simulink library "halout"  (R2021b)
settings: Solver=VariableStepAuto  StartTime=0.0  StopTime=10.0  RelTol=1e-3
undefined symbols (not defined in the file): C_TASK_5MS_S, KHAL_CAN1TxReq_flg, KHAL_CAN2TxReq_flg, KHAL_CAN3TxReq_flg, KHAL_CAN4TxReq_flg, KHAL_CAN5TxReq_flg, KHAL_CAN6TxReq_flg, KHAL_CAN7TxReq_flg, TRUE
libraries: FVT_lib x65, simulink x6
(part 3 of 6)

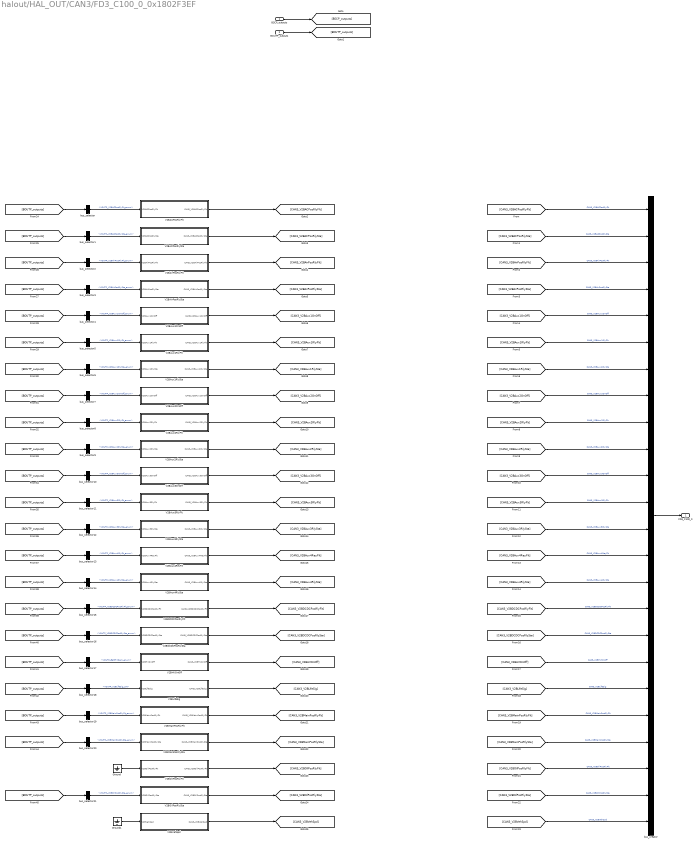
== system halout/HAL_OUT/CAN3/FD3_C100_0_0x1802F3EF ==
  BSCP_outputs : Inport  OutDataTypeStr=Bus: BSCP_outputs
  BOUTP_outputs : Inport  Port=2  OutDataTypeStr=Bus: BOUTP_outputs
  Ground : Ground
  Ground1 : Ground
  V2BACPosRlyFlt : Subsystem
  V2BACPosRlySta : Subsystem
  V2BAirPosRlyFlt : Subsystem
  V2BAirPosRlySta : Subsystem
  V2BAux1OnOff : Subsystem
  V2BAux1RlyFlt : Subsystem
  V2BAux1RlySta : Subsystem
  V2BAux2OnOff : Subsystem
  V2BAux2RlyFlt : Subsystem
  V2BAux2RlySta : Subsystem
  V2BAux3OnOff : Subsystem
  V2BAux3RlyFlt : Subsystem
  V2BAux3RlySta : Subsystem
  V2BAux4ReyFlt : Subsystem
  V2BAux4RlySta : Subsystem
  V2BDCDCPosRlyFlt : Subsystem
  V2BDCDCPosRlySta : Subsystem
  V2BHVOnOff : Subsystem
  V2BLifeSig : Subsystem
  V2BMainPosRlyFlt : Subsystem
  V2BMainPosRlySta : Subsystem
  V2BOilPosRlyFlt : Subsystem
  V2BOilPosRlySta : Subsystem
  V2BVehSpd : Subsystem
  bus_creator : BusCreator  Inputs=24  OutDataTypeStr=Bus: DT_CAN3_SG_FD3_C100_0  NonVirtualBus=on
  bus_selector : BusSelector  OutputSignals=VOUTP_V2BACPosRlyFit_enum
  bus_selector1 : BusSelector  OutputSignals=VOUTP_V2BACPosRlySta_enum
  bus_selector10 : BusSelector  OutputSignals=VOUTP_V2BAux3OnOff_enum
  bus_selector11 : BusSelector  OutputSignals=VOUTP_V2BAux3RlyFit_enum
  bus_selector12 : BusSelector  OutputSignals=VOUTP_V2BAux3RlySta_enum
  bus_selector13 : BusSelector  OutputSignals=VOUTP_V2BAux4RlyFit_enum
  bus_selector14 : BusSelector  OutputSignals=VOUTP_V2BAux4RlySta_enum
  bus_selector15 : BusSelector  OutputSignals=VOUTP_V2BDCDCPosRlyFit_enum
  bus_selector16 : BusSelector  OutputSignals=VOUTP_V2BDCDCPosRlySta_enum
  bus_selector17 : BusSelector  OutputSignals=VOUTP_BattHVDem_enum
  bus_selector18 : BusSelector  OutputSignals=VOUTP_V2BLifeSig_cnt
  bus_selector19 : BusSelector  OutputSignals=VOUTP_V2BMainPosRlyFit_enum
  bus_selector2 : BusSelector  OutputSignals=VOUTP_V2BAirPosRlyFit_enum
  bus_selector20 : BusSelector  OutputSignals=VOUTP_V2BMainPosRlySta_enum
  bus_selector21 : BusSelector  OutputSignals=VOUTP_V2BOilPosRlySta_enum
  bus_selector3 : BusSelector  OutputSignals=VOUTP_V2BAirPosRlySta_enum
  bus_selector4 : BusSelector  OutputSignals=VOUTP_V2BAux1OnOff_enum
  bus_selector5 : BusSelector  OutputSignals=VOUTP_V2BAux1RlyFit_enum
  bus_selector6 : BusSelector  OutputSignals=VOUTP_V2BAux1RlySta_enum
  bus_selector7 : BusSelector  OutputSignals=VOUTP_V2BAux2OnOff_enum
  bus_selector8 : BusSelector  OutputSignals=VOUTP_V2BAux2RlyFit_enum
  bus_selector9 : BusSelector  OutputSignals=VOUTP_V2BAux2RlySta_enum
  FD3_C100_0 : Outport
  wires:
  BSCP_outputs/1 -> [BSCP_outputs]
  BOUTP_outputs/1 -> [BOUTP_outputs]
  [CAN3_V2BACPosRlyFlt] -> bus_creator/1  "CAN3_V2BACPosRlyFlt"
  [CAN3_V2BACPosRlySta] -> bus_creator/2  "CAN3_V2BACPosRlySta"
  [CAN3_V2BAirPosRlyFlt] -> bus_creator/3  "CAN3_V2BAirPosRlyFlt"
  [CAN3_V2BAirPosRlySta] -> bus_creator/4  "CAN3_V2BAirPosRlySta"
  [CAN3_V2BAux1OnOff] -> bus_creator/5  "CAN3_V2BAux1OnOff"
  [CAN3_V2BAux1RlyFlt] -> bus_creator/6  "CAN3_V2BAux1RlyFlt"
  [CAN3_V2BAux1RlySta] -> bus_creator/7  "CAN3_V2BAux1RlySta"
  [CAN3_V2BAux2OnOff] -> bus_creator/8  "CAN3_V2BAux2OnOff"
  [CAN3_V2BAux2RlyFlt] -> bus_creator/9  "CAN3_V2BAux2RlyFlt"
  [CAN3_V2BAux2RlySta] -> bus_creator/10  "CAN3_V2BAux2RlySta"
  [CAN3_V2BAux3OnOff] -> bus_creator/11  "CAN3_V2BAux3OnOff"
  [CAN3_V2BAux3RlyFlt] -> bus_creator/12  "CAN3_V2BAux3RlyFlt"
  [CAN3_V2BAux3RlySta] -> bus_creator/13  "CAN3_V2BAux3RlySta"
  [CAN3_V2BAux4ReyFlt] -> bus_creator/14  "CAN3_V2BAux4ReyFlt"
  [CAN3_V2BAux4RlySta] -> bus_creator/15  "CAN3_V2BAux4RlySta"
  [CAN3_V2BDCDCPosRlyFlt] -> bus_creator/16  "CAN3_V2BDCDCPosRlyFlt"
  [CAN3_V2BDCDCPosRlySta] -> bus_creator/17  "CAN3_V2BDCDCPosRlySta"
  [CAN3_V2BHVOnOff] -> bus_creator/18  "CAN3_V2BHVOnOff"
  [CAN3_V2BLifeSig] -> bus_creator/19  "CAN3_V2BLifeSig"
  [CAN3_V2BMainPosRlyFlt] -> bus_creator/20  "CAN3_V2BMainPosRlyFlt"
  [CAN3_V2BMainPosRlySta] -> bus_creator/21  "CAN3_V2BMainPosRlySta"
  [CAN3_V2BOilPosRlyFlt] -> bus_creator/22  "CAN3_V2BOilPosRlyFlt"
  [CAN3_V2BOilPosRlySta] -> bus_creator/23  "CAN3_V2BOilPosRlySta"
  [CAN3_V2BVehSpd] -> bus_creator/24  "CAN3_V2BVehSpd"
  bus_creator/1 -> FD3_C100_0/1
  V2BACPosRlyFlt/1(CAN3_V2BACPosRlyFlt) -> [CAN3_V2BACPosRlyFlt]
  V2BACPosRlySta/1(CAN3_V2BACPosRlySta) -> [CAN3_V2BACPosRlySta]
  V2BAirPosRlyFlt/1(CAN3_V2BAirPosRlyFlt) -> [CAN3_V2BAirPosRlyFlt]
  V2BAirPosRlySta/1(CAN3_V2BAirPosRlySta) -> [CAN3_V2BAirPosRlySta]
  V2BAux1OnOff/1(CAN3_V2BAux1OnOff) -> [CAN3_V2BAux1OnOff]
  V2BAux1RlyFlt/1(CAN3_V2BAux1RlyFlt) -> [CAN3_V2BAux1RlyFlt]
  V2BAux1RlySta/1(CAN3_V2BAux1RlySta) -> [CAN3_V2BAux1RlySta]
  V2BAux2OnOff/1(CAN3_V2BAux2OnOff) -> [CAN3_V2BAux2OnOff]
  V2BAux2RlyFlt/1(CAN3_V2BAux2RlyFlt) -> [CAN3_V2BAux2RlyFlt]
  V2BAux2RlySta/1(CAN3_V2BAux2RlySta) -> [CAN3_V2BAux2RlySta]
  V2BAux3OnOff/1(CAN3_V2BAux3OnOff) -> [CAN3_V2BAux3OnOff]
  V2BAux3RlyFlt/1(CAN3_V2BAux3RlyFlt) -> [CAN3_V2BAux3RlyFlt]
  V2BAux3RlySta/1(CAN3_V2BAux3RlySta) -> [CAN3_V2BAux3RlySta]
  V2BAux4ReyFlt/1(CAN3_V2BAux4ReyFlt) -> [CAN3_V2BAux4ReyFlt]
  V2BAux4RlySta/1(CAN3_V2BAux4RlySta) -> [CAN3_V2BAux4RlySta]
  V2BDCDCPosRlyFlt/1(CAN3_V2BDCDCPosRlyFlt) -> [CAN3_V2BDCDCPosRlyFlt]
  V2BDCDCPosRlySta/1(CAN3_V2BDCDCPosRlySta) -> [CAN3_V2BDCDCPosRlySta]
  V2BHVOnOff/1(CAN3_V2BHVOnOff) -> [CAN3_V2BHVOnOff]
  V2BLifeSig/1(CAN3_V2BLifeSig) -> [CAN3_V2BLifeSig]
  V2BMainPosRlyFlt/1(CAN3_V2BMainPosRlyFlt) -> [CAN3_V2BMainPosRlyFlt]
  V2BMainPosRlySta/1(CAN3_V2BMainPosRlySta) -> [CAN3_V2BMainPosRlySta]
  V2BOilPosRlyFlt/1(CAN3_V2BOilPosRlyFlt) -> [CAN3_V2BOilPosRlyFlt]
  V2BOilPosRlySta/1(CAN3_V2BOilPosRlySta) -> [CAN3_V2BOilPosRlySta]
  V2BVehSpd/1(CAN3_V2BVehSpd) -> [CAN3_V2BVehSpd]
  bus_selector/1 -> V2BACPosRlyFlt/1(V2BACPosRlyFlt)  "<VOUTP_V2BACPosRlyFit_enum>"
  [BOUTP_outputs] -> bus_selector/1
  bus_selector1/1 -> V2BACPosRlySta/1(V2BACPosRlySta)  "<VOUTP_V2BACPosRlySta_enum>"
  [BOUTP_outputs] -> bus_selector1/1
  bus_selector2/1 -> V2BAirPosRlyFlt/1(V2BAirPosRlyFlt)  "<VOUTP_V2BAirPosRlyFit_enum>"
  [BOUTP_outputs] -> bus_selector2/1
  bus_selector3/1 -> V2BAirPosRlySta/1(V2BAirPosRlySta)  "<VOUTP_V2BAirPosRlySta_enum>"
  [BOUTP_outputs] -> bus_selector3/1
  bus_selector4/1 -> V2BAux1OnOff/1(V2BAux1OnOff)  "<VOUTP_V2BAux1OnOff_enum>"
  [BOUTP_outputs] -> bus_selector4/1
  bus_selector5/1 -> V2BAux1RlyFlt/1(V2BAux1RlyFlt)  "<VOUTP_V2BAux1RlyFit_enum>"
  [BOUTP_outputs] -> bus_selector5/1
  bus_selector6/1 -> V2BAux1RlySta/1(V2BAux1RlySta)  "<VOUTP_V2BAux1RlySta_enum>"
  [BOUTP_outputs] -> bus_selector6/1
  bus_selector7/1 -> V2BAux2OnOff/1(V2BAux2OnOff)  "<VOUTP_V2BAux2OnOff_enum>"
  [BOUTP_outputs] -> bus_selector7/1
  bus_selector8/1 -> V2BAux2RlyFlt/1(V2BAux2RlyFlt)  "<VOUTP_V2BAux2RlyFit_enum>"
  [BOUTP_outputs] -> bus_selector8/1
  bus_selector9/1 -> V2BAux2RlySta/1(V2BAux2RlySta)  "<VOUTP_V2BAux2RlySta_enum>"
  [BOUTP_outputs] -> bus_selector9/1
  bus_selector10/1 -> V2BAux3OnOff/1(V2BAux3OnOff)  "<VOUTP_V2BAux3OnOff_enum>"
  [BOUTP_outputs] -> bus_selector10/1
  bus_selector11/1 -> V2BAux3RlyFlt/1(V2BAux3RlyFlt)  "<VOUTP_V2BAux3RlyFit_enum>"
  [BOUTP_outputs] -> bus_selector11/1
  bus_selector12/1 -> V2BAux3RlySta/1(V2BAux3RlySta)  "<VOUTP_V2BAux3RlySta_enum>"
  [BOUTP_outputs] -> bus_selector12/1
  bus_selector13/1 -> V2BAux4ReyFlt/1(V2BAux4ReyFlt)  "<VOUTP_V2BAux4RlyFit_enum>"
  [BOUTP_outputs] -> bus_selector13/1
  bus_selector14/1 -> V2BAux4RlySta/1(V2BAux4RlySta)  "<VOUTP_V2BAux4RlySta_enum>"
  [BOUTP_outputs] -> bus_selector14/1
  bus_selector15/1 -> V2BDCDCPosRlyFlt/1(V2BDCDCPosRlyFlt)  "<VOUTP_V2BDCDCPosRlyFit_enum>"
  [BOUTP_outputs] -> bus_selector15/1
  bus_selector16/1 -> V2BDCDCPosRlySta/1(V2BDCDCPosRlySta)  "<VOUTP_V2BDCDCPosRlySta_enum>"
  [BOUTP_outputs] -> bus_selector16/1
  bus_selector17/1 -> V2BHVOnOff/1(V2BHVOnOff)  "<VOUTP_BattHVDem_enum>"
  [BOUTP_outputs] -> bus_selector17/1
  bus_selector18/1 -> V2BLifeSig/1(V2BLifeSig)  "<VOUTP_V2BLifeSig_cnt>"
  [BOUTP_outputs] -> bus_selector18/1
  bus_selector19/1 -> V2BMainPosRlyFlt/1(V2BMainPosRlyFlt)  "<VOUTP_V2BMainPosRlyFit_enum>"
  [BOUTP_outputs] -> bus_selector19/1
  bus_selector20/1 -> V2BMainPosRlySta/1(V2BMainPosRlySta)  "<VOUTP_V2BMainPosRlySta_enum>"
  [BOUTP_outputs] -> bus_selector20/1
  Ground/1 -> V2BOilPosRlyFlt/1(V2BOilPosRlyFlt)
  bus_selector21/1 -> V2BOilPosRlySta/1(V2BOilPosRlySta)  "<VOUTP_V2BOilPosRlySta_enum>"
  [BOUTP_outputs] -> bus_selector21/1
  Ground1/1 -> V2BVehSpd/1(V2BVehSpd)

== system halout/HAL_OUT/CAN3/FD3_C10_0_0xCF101D0 ==
  BSCP_outputs : Inport  OutDataTypeStr=Bus: BSCP_outputs
  BOUTP_outputs : Inport  Port=2  OutDataTypeStr=Bus: BOUTP_outputs
  DCDCRlyEn : Subsystem
  EACRlyEn : Subsystem
  EHPSRlyEn : Subsystem
  Ground : Ground
  MCUHVPwrOnOffReq : Subsystem
  VCULife1 : Subsystem
  bus_creator : BusCreator  Inputs=5  OutDataTypeStr=Bus: DT_CAN3_SG_FD3_C10_0  NonVirtualBus=on
  bus_selector : BusSelector  OutputSignals=VOUTP_DCDCRlyDem_enum
  bus_selector1 : BusSelector  OutputSignals=VOUTP_EHPSRlyDem_enum
  bus_selector2 : BusSelector  OutputSignals=VOUTP_MCUHVLoopDem_enum
  bus_selector3 : BusSelector  OutputSignals=VOUTP_VCULife1_cnt
  FD3_C10_0 : Outport
  wires:
  BSCP_outputs/1 -> [BSCP_outputs]
  BOUTP_outputs/1 -> [BOUTP_outputs]
  [CAN3_DCDCRlyEn] -> bus_creator/1  "CAN3_DCDCRlyEn"
  [CAN3_EACRlyEn] -> bus_creator/2  "CAN3_EACRlyEn"
  [CAN3_EHPSRlyEn] -> bus_creator/3  "CAN3_EHPSRlyEn"
  [CAN3_MCUHVPwrOnOffReq] -> bus_creator/4  "CAN3_MCUHVPwrOnOffReq"
  [CAN3_VCULife1] -> bus_creator/5  "CAN3_VCULife1"
  bus_creator/1 -> FD3_C10_0/1
  DCDCRlyEn/1(CAN3_DCDCRlyEn) -> [CAN3_DCDCRlyEn]
  EACRlyEn/1(CAN3_EACRlyEn) -> [CAN3_EACRlyEn]
  EHPSRlyEn/1(CAN3_EHPSRlyEn) -> [CAN3_EHPSRlyEn]
  MCUHVPwrOnOffReq/1(CAN3_MCUHVPwrOnOffReq) -> [CAN3_MCUHVPwrOnOffReq]
  VCULife1/1(CAN3_VCULife1) -> [CAN3_VCULife1]
  bus_selector/1 -> DCDCRlyEn/1(DCDCRlyEn)  "<VOUTP_DCDCRlyDem_enum>"
  [BOUTP_outputs] -> bus_selector/1
  Ground/1 -> EACRlyEn/1(EACRlyEn)
  bus_selector1/1 -> EHPSRlyEn/1(EHPSRlyEn)  "<VOUTP_EHPSRlyDem_enum>"
  [BOUTP_outputs] -> bus_selector1/1
  bus_selector2/1 -> MCUHVPwrOnOffReq/1(MCUHVPwrOnOffReq)  "<VOUTP_MCUHVLoopDem_enum>"
  [BOUTP_outputs] -> bus_selector2/1
  bus_selector3/1 -> VCULife1/1(VCULife1)  "<VOUTP_VCULife1_cnt>"
  [BOUTP_outputs] -> bus_selector3/1

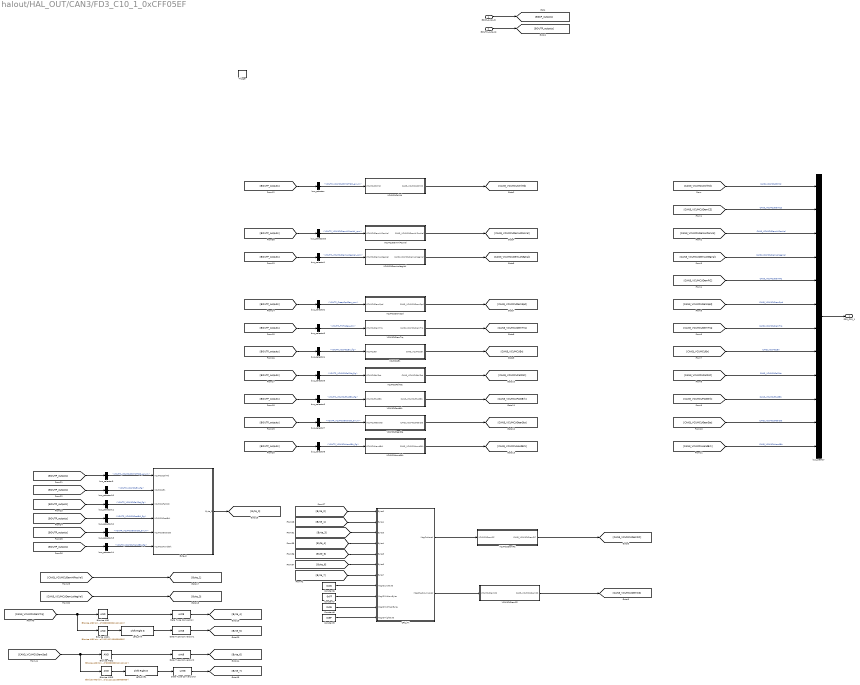
== system halout/HAL_OUT/CAN3/FD3_C10_1_0xCFF05EF ==
  BSCP_outputs : Inport  OutDataTypeStr=Bus: BSCP_outputs
  BOUTP_outputs : Inport  Port=2  OutDataTypeStr=Bus: BOUTP_outputs
  Trigger : TriggerPort  TriggerType=function-call  VariantControl=(inherit)
  Bitwise AND : simulink/Logic and Bit Operations/Bitwise Operator  logicop=AND  UseBitMask=on  BitMask=bin2dec('0000000011111111')  BitMaskRealWorld=Stored Integer
  Bitwise AND1 : simulink/Logic and Bit Operations/Bitwise Operator  logicop=AND  UseBitMask=on  BitMask=bin2dec('1111111100000000')  BitMaskRealWorld=Stored Integer
  Bitwise AND2 : simulink/Logic and Bit Operations/Bitwise Operator  logicop=AND  UseBitMask=on  BitMask=bin2dec('0000000011111111')  BitMaskRealWorld=Stored Integer
  Bitwise AND3 : simulink/Logic and Bit Operations/Bitwise Operator  logicop=AND  UseBitMask=on  BitMask=bin2dec('1111111100000000')  BitMaskRealWorld=Stored Integer
  Byte_0 : Subsystem
  CRC_TX : Subsystem
  Constant6 : Constant  Value=0x0C
  Constant7 : Constant  Value=0xFF
  Constant8 : Constant  Value=0x05
  Constant9 : Constant  Value=0xEF
  Data Type Conversion{,1..3} (4 alike) : DataTypeConversion  OutDataTypeStr=uint8
  Left_shift : ArithShift  BitShiftNumber=8  BitShiftDirection=Right
  Left_shift1 : ArithShift  BitShiftNumber=8  BitShiftDirection=Right
  VCUMCUCtrlMd : Subsystem
  VCUMCUDemCS : Subsystem
  VCUMCUDemHiPosVal : Subsystem
  VCUMCUDemLoNegVal : Subsystem
  VCUMCUDemRC : Subsystem
  VCUMCUDemSpd : Subsystem
  VCUMCUDemTrq : Subsystem
  VCUMCUEn : Subsystem
  VCUMCUFailRst : Subsystem
  VCUMCUFootBrk : Subsystem
  VCUMCUGearSta : Subsystem
  VCUMCUHandBrk : Subsystem
  bus_creator : BusCreator  Inputs=12  OutDataTypeStr=Bus: DT_CAN3_SG_FD3_C10_1  NonVirtualBus=on
  bus_selector : BusSelector  OutputSignals=VOUTP_VCUMCUCtrlMdTQD_enum
  bus_selector1 : BusSelector  OutputSignals=VOUTP_VCUMCUDemLoNegVal_rpm
  bus_selector10 : BusSelector  OutputSignals=VOUTP_VCUMCUEn_flg
  bus_selector11 : BusSelector  OutputSignals=VOUTP_VCUMCUFailRst_flg
  bus_selector12 : BusSelector  OutputSignals=VOUTP_VCUMCUFootBrk_flg
  bus_selector13 : BusSelector  OutputSignals=VOUTP_VCUMCUGearSta_enum
  bus_selector14 : BusSelector  OutputSignals=VOUTP_VCUMCUHandBrk_flg
  bus_selector2 : BusSelector  OutputSignals=VOUTP_CreepSpdReq_rpm
  bus_selector20 : BusSelector  OutputSignals=VOUTP_VCUMCUDemHiPosVal_rpm
  bus_selector3 : BusSelector  OutputSignals=VOUTP_TMTqReq_Nm
  bus_selector4 : BusSelector  OutputSignals=VOUTP_VCUMCUEn_flg
  bus_selector5 : BusSelector  OutputSignals=VOUTP_VCUMCUFailRst_flg
  bus_selector6 : BusSelector  OutputSignals=VOUTP_VCUMCUFootBrk_flg
  bus_selector7 : BusSelector  OutputSignals=VOUTP_VCUMCUGearSta_enum
  bus_selector8 : BusSelector  OutputSignals=VOUTP_VCUMCUHandBrk_flg
  bus_selector9 : BusSelector  OutputSignals=VOUTP_VCUMCUCtrlMdTQD_enum
  FD3_C10_1 : Outport
  wires:
  BSCP_outputs/1 -> [BSCP_outputs]
  BOUTP_outputs/1 -> [BOUTP_outputs]
  [CAN3_VCUMCUCtrlMd] -> bus_creator/1  "CAN3_VCUMCUCtrlMd"
  [CAN3_VCUMCUDemCS] -> bus_creator/2  "CAN3_VCUMCUDemCS"
  [CAN3_VCUMCUDemHiPosVal] -> bus_creator/3  "CAN3_VCUMCUDemHiPosVal"
  [CAN3_VCUMCUDemLoNegVal] -> bus_creator/4  "CAN3_VCUMCUDemLoNegVal"
  [CAN3_VCUMCUDemRC] -> bus_creator/5  "CAN3_VCUMCUDemRC"
  [CAN3_VCUMCUDemSpd] -> bus_creator/6  "CAN3_VCUMCUDemSpd"
  [CAN3_VCUMCUDemTrq] -> bus_creator/7  "CAN3_VCUMCUDemTrq"
  [CAN3_VCUMCUEn] -> bus_creator/8  "CAN3_VCUMCUEn"
  [CAN3_VCUMCUFailRst] -> bus_creator/9  "CAN3_VCUMCUFailRst"
  [CAN3_VCUMCUFootBrk] -> bus_creator/10  "CAN3_VCUMCUFootBrk"
  [CAN3_VCUMCUGearSta] -> bus_creator/11  "CAN3_VCUMCUGearSta"
  [CAN3_VCUMCUHandBrk] -> bus_creator/12  "CAN3_VCUMCUHandBrk"
  bus_creator/1 -> FD3_C10_1/1
  VCUMCUCtrlMd/1(CAN3_VCUMCUCtrlMd) -> [CAN3_VCUMCUCtrlMd]
  VCUMCUDemCS/1(CAN3_VCUMCUDemCS) -> [CAN3_VCUMCUDemCS]
  VCUMCUDemHiPosVal/1(CAN3_VCUMCUDemHiPosVal) -> [CAN3_VCUMCUDemHiPosVal]
  VCUMCUDemLoNegVal/1(CAN3_VCUMCUDemLoNegVal) -> [CAN3_VCUMCUDemLoNegVal]
  VCUMCUDemRC/1(CAN3_VCUMCUDemRC) -> [CAN3_VCUMCUDemRC]
  VCUMCUDemSpd/1(CAN3_VCUMCUDemSpd) -> [CAN3_VCUMCUDemSpd]
  VCUMCUDemTrq/1(CAN3_VCUMCUDemTrq) -> [CAN3_VCUMCUDemTrq]
  VCUMCUEn/1(CAN3_VCUMCUEn) -> [CAN3_VCUMCUEn]
  VCUMCUFailRst/1(CAN3_VCUMCUFailRst) -> [CAN3_VCUMCUFailRst]
  VCUMCUFootBrk/1(CAN3_VCUMCUFootBrk) -> [CAN3_VCUMCUFootBrk]
  VCUMCUGearSta/1(CAN3_VCUMCUGearSta) -> [CAN3_VCUMCUGearSta]
  VCUMCUHandBrk/1(CAN3_VCUMCUHandBrk) -> [CAN3_VCUMCUHandBrk]
  bus_selector/1 -> VCUMCUCtrlMd/1(VCUMCUCtrlMd)  "<VOUTP_VCUMCUCtrlMdTQD_enum>"
  [BOUTP_outputs] -> bus_selector/1
  CRC_TX/2(MsgChecksumLocal) -> VCUMCUDemCS/1(VCUMCUDemCS)
  bus_selector1/1 -> VCUMCUDemLoNegVal/1(VCUMCUDemLoNegVal)  "<VOUTP_VCUMCUDemLoNegVal_rpm>"
  [BOUTP_outputs] -> bus_selector1/1
  CRC_TX/1(MsgCntLocal) -> VCUMCUDemRC/1(VCUMCUDemRC)
  bus_selector2/1 -> VCUMCUDemSpd/1(VCUMCUDemSpd)  "<VOUTP_CreepSpdReq_rpm>"
  [BOUTP_outputs] -> bus_selector2/1
  bus_selector3/1 -> VCUMCUDemTrq/1(VCUMCUDemTrq)  "<VOUTP_TMTqReq_Nm>"
  [BOUTP_outputs] -> bus_selector3/1
  bus_selector4/1 -> VCUMCUEn/1(VCUMCUEn)  "<VOUTP_VCUMCUEn_flg>"
  [BOUTP_outputs] -> bus_selector4/1
  bus_selector5/1 -> VCUMCUFailRst/1(VCUMCUFailRst)  "<VOUTP_VCUMCUFailRst_flg>"
  [BOUTP_outputs] -> bus_selector5/1
  bus_selector6/1 -> VCUMCUFootBrk/1(VCUMCUFootBrk)  "<VOUTP_VCUMCUFootBrk_flg>"
  [BOUTP_outputs] -> bus_selector6/1
  bus_selector7/1 -> VCUMCUGearSta/1(VCUMCUGearSta)  "<VOUTP_VCUMCUGearSta_enum>"
  [BOUTP_outputs] -> bus_selector7/1
  bus_selector8/1 -> VCUMCUHandBrk/1(VCUMCUHandBrk)  "<VOUTP_VCUMCUHandBrk_flg>"
  [BOUTP_outputs] -> bus_selector8/1
  Constant6/1 -> CRC_TX/8(MsgIDLowByte)
  Constant9/1 -> CRC_TX/11(MsgIDHighByte)
  Constant7/1 -> CRC_TX/9(MsgIDMidLowByte)
  Constant8/1 -> CRC_TX/10(MsgIDMidHighByte)
  [BOUTP_outputs] -> bus_selector14/1
  bus_selector10/1 -> Byte_0/2(VCUMCUEn)  "<VOUTP_VCUMCUEn_flg>"
  bus_selector13/1 -> Byte_0/5(VCUMCUGearSta)  "<VOUTP_VCUMCUGearSta_enum>"
  [BOUTP_outputs] -> bus_selector12/1
  [BOUTP_outputs] -> bus_selector11/1
  bus_selector14/1 -> Byte_0/6(VCUMCUHandBrk)  "<VOUTP_VCUMCUHandBrk_flg>"
  [BOUTP_outputs] -> bus_selector10/1
  bus_selector11/1 -> Byte_0/3(VCUMCUFailRst)  "<VOUTP_VCUMCUFailRst_flg>"
  Byte_0/1(Byte_0) -> [Byte_0]
  bus_selector9/1 -> Byte_0/1(VCUMCUCtrlMd)  "<VOUTP_VCUMCUCtrlMdTQD_enum>"
  [BOUTP_outputs] -> bus_selector9/1
  [BOUTP_outputs] -> bus_selector13/1
  bus_selector12/1 -> Byte_0/4(VCUMCUFootBrk)  "<VOUTP_VCUMCUFootBrk_flg>"
  [Byte_0] -> CRC_TX/1(Byte0)
  [CAN3_VCUMCUDemHiPosVal] -> [Byte_1]
  [Byte_1] -> CRC_TX/2(Byte1)
  [Byte_3] -> CRC_TX/3(Byte3)
  [Byte_7] -> CRC_TX/7(Byte7)
  [Byte_4] -> CRC_TX/4(Byte4)
  [Byte_5] -> CRC_TX/5(Byte5)
  [Byte_6] -> CRC_TX/6(Byte6)
  [BOUTP_outputs] -> bus_selector20/1
  bus_selector20/1 -> VCUMCUDemHiPosVal/1(VCUMCUDemHiPosVal)  "<VOUTP_VCUMCUDemHiPosVal_rpm>"
  [CAN3_VCUMCUDemTrq] -> Bitwise AND1/1, Bitwise AND/1
  Bitwise AND/1 -> Data Type Conversion/1
  Bitwise AND1/1 -> Left_shift/1
  Left_shift/1 -> Data Type Conversion1/1
  Bitwise AND3/1 -> Left_shift1/1
  [CAN3_VCUMCUDemSpd] -> Bitwise AND3/1, Bitwise AND2/1
  Bitwise AND2/1 -> Data Type Conversion2/1
  Left_shift1/1 -> Data Type Conversion3/1
  [CAN3_VCUMCUDemLoNegVal] -> [Byte_3]
  Data Type Conversion1/1 -> [Byte_5]
  Data Type Conversion/1 -> [Byte_4]
  Data Type Conversion2/1 -> [Byte_6]
  Data Type Conversion3/1 -> [Byte_7]

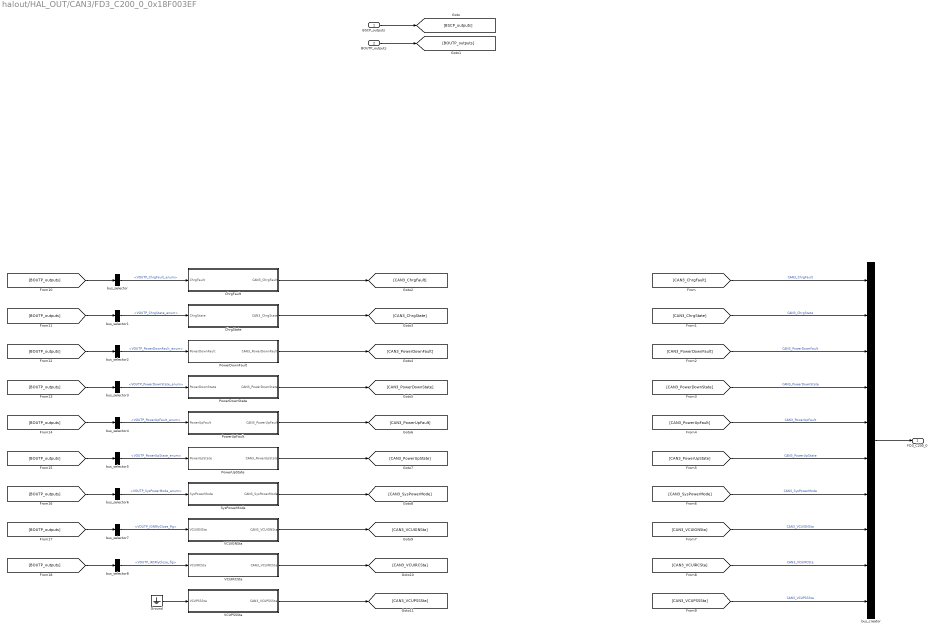
== system halout/HAL_OUT/CAN3/FD3_C200_0_0x18F003EF ==
  BSCP_outputs : Inport  OutDataTypeStr=Bus: BSCP_outputs
  BOUTP_outputs : Inport  Port=2  OutDataTypeStr=Bus: BOUTP_outputs
  ChrgFault : Subsystem
  ChrgState : Subsystem
  Ground : Ground
  PowerDownFault : Subsystem
  PowerDownState : Subsystem
  PowerUpFault : Subsystem
  PowerUpState : Subsystem
  SysPowerMode : Subsystem
  VCUIGNSta : Subsystem
  VCUIRCSta : Subsystem
  VCUPSSSta : Subsystem
  bus_creator : BusCreator  Inputs=10  OutDataTypeStr=Bus: DT_CAN3_SG_FD3_C200_0  NonVirtualBus=on
  bus_selector : BusSelector  OutputSignals=VOUTP_ChrgFault_enum
  bus_selector1 : BusSelector  OutputSignals=VOUTP_ChrgState_enum
  bus_selector2 : BusSelector  OutputSignals=VOUTP_PowerDownFault_enum
  bus_selector3 : BusSelector  OutputSignals=VOUTP_PowerDownState_enum
  bus_selector4 : BusSelector  OutputSignals=VOUTP_PowerUpFault_enum
  bus_selector5 : BusSelector  OutputSignals=VOUTP_PowerUpState_enum
  bus_selector6 : BusSelector  OutputSignals=VOUTP_SysPowerMode_enum
  bus_selector7 : BusSelector  OutputSignals=VOUTP_IGNRlyClose_flg
  bus_selector8 : BusSelector  OutputSignals=VOUTP_IRCRlyClose_flg
  FD3_C200_0 : Outport
  wires:
  BSCP_outputs/1 -> [BSCP_outputs]
  BOUTP_outputs/1 -> [BOUTP_outputs]
  [CAN3_ChrgFault] -> bus_creator/1  "CAN3_ChrgFault"
  [CAN3_ChrgState] -> bus_creator/2  "CAN3_ChrgState"
  [CAN3_PowerDownFault] -> bus_creator/3  "CAN3_PowerDownFault"
  [CAN3_PowerDownState] -> bus_creator/4  "CAN3_PowerDownState"
  [CAN3_PowerUpFault] -> bus_creator/5  "CAN3_PowerUpFault"
  [CAN3_PowerUpState] -> bus_creator/6  "CAN3_PowerUpState"
  [CAN3_SysPowerMode] -> bus_creator/7  "CAN3_SysPowerMode"
  [CAN3_VCUIGNSta] -> bus_creator/8  "CAN3_VCUIGNSta"
  [CAN3_VCUIRCSta] -> bus_creator/9  "CAN3_VCUIRCSta"
  [CAN3_VCUPSSSta] -> bus_creator/10  "CAN3_VCUPSSSta"
  bus_creator/1 -> FD3_C200_0/1
  ChrgFault/1(CAN3_ChrgFault) -> [CAN3_ChrgFault]
  ChrgState/1(CAN3_ChrgState) -> [CAN3_ChrgState]
  PowerDownFault/1(CAN3_PowerDownFault) -> [CAN3_PowerDownFault]
  PowerDownState/1(CAN3_PowerDownState) -> [CAN3_PowerDownState]
  PowerUpFault/1(CAN3_PowerUpFault) -> [CAN3_PowerUpFault]
  PowerUpState/1(CAN3_PowerUpState) -> [CAN3_PowerUpState]
  SysPowerMode/1(CAN3_SysPowerMode) -> [CAN3_SysPowerMode]
  VCUIGNSta/1(CAN3_VCUIGNSta) -> [CAN3_VCUIGNSta]
  VCUIRCSta/1(CAN3_VCUIRCSta) -> [CAN3_VCUIRCSta]
  VCUPSSSta/1(CAN3_VCUPSSSta) -> [CAN3_VCUPSSSta]
  bus_selector/1 -> ChrgFault/1(ChrgFault)  "<VOUTP_ChrgFault_enum>"
  [BOUTP_outputs] -> bus_selector/1
  bus_selector1/1 -> ChrgState/1(ChrgState)  "<VOUTP_ChrgState_enum>"
  [BOUTP_outputs] -> bus_selector1/1
  bus_selector2/1 -> PowerDownFault/1(PowerDownFault)  "<VOUTP_PowerDownFault_enum>"
  [BOUTP_outputs] -> bus_selector2/1
  bus_selector3/1 -> PowerDownState/1(PowerDownState)  "<VOUTP_PowerDownState_enum>"
  [BOUTP_outputs] -> bus_selector3/1
  bus_selector4/1 -> PowerUpFault/1(PowerUpFault)  "<VOUTP_PowerUpFault_enum>"
  [BOUTP_outputs] -> bus_selector4/1
  bus_selector5/1 -> PowerUpState/1(PowerUpState)  "<VOUTP_PowerUpState_enum>"
  [BOUTP_outputs] -> bus_selector5/1
  bus_selector6/1 -> SysPowerMode/1(SysPowerMode)  "<VOUTP_SysPowerMode_enum>"
  [BOUTP_outputs] -> bus_selector6/1
  bus_selector7/1 -> VCUIGNSta/1(VCUIGNSta)  "<VOUTP_IGNRlyClose_flg>"
  [BOUTP_outputs] -> bus_selector7/1
  bus_selector8/1 -> VCUIRCSta/1(VCUIRCSta)  "<VOUTP_IRCRlyClose_flg>"
  [BOUTP_outputs] -> bus_selector8/1
  Ground/1 -> VCUPSSSta/1(VCUPSSSta)

== system halout/HAL_OUT/CAN3/FD3_C200_1_0x18F001EF ==
  BSCP_outputs : Inport  OutDataTypeStr=Bus: BSCP_outputs
  BOUTP_outputs : Inport  Port=2  OutDataTypeStr=Bus: BOUTP_outputs
  FDCTHCMEWPPEReqCmd : Subsystem
  bus_creator : BusCreator  Inputs=1  OutDataTypeStr=Bus: DT_CAN3_SG_FD3_C200_1  NonVirtualBus=on
  bus_selector : BusSelector  OutputSignals=VOUTP_EWPPEReq_rpm
  FD3_C200_1 : Outport
  wires:
  BSCP_outputs/1 -> [BSCP_outputs]
  BOUTP_outputs/1 -> [BOUTP_outputs]
  [CAN3_FDC_THCM_EWPPEReq_Cmd] -> bus_creator/1  "CAN3_FDC_THCM_EWPPEReq_Cmd"
  bus_creator/1 -> FD3_C200_1/1
  FDCTHCMEWPPEReqCmd/1(CAN3_FDC_THCM_EWPPEReq_Cmd) -> [CAN3_FDC_THCM_EWPPEReq_Cmd]
  bus_selector/1 -> FDCTHCMEWPPEReqCmd/1(FDCTHCMEWPPEReqCmd)  "<VOUTP_EWPPEReq_rpm>"
  [BOUTP_outputs] -> bus_selector/1

== system halout/HAL_OUT/CAN3/FD3_VCU2_Tx ==
  TxReq : Inport
  Chart : Stateflow chart  TreatAsAtomicUnit=on
  Constant : Constant  Value=C_TASK_5MS_S
  Constant3 : Constant  Value=CycleTime
  Data Type Conversion : DataTypeConversion  OutDataTypeStr=uint16
  Divide : Product  Inputs=*/
  Gain : Gain  Gain=0.001
  TxTrigger : Outport
  wires:
  Constant/1 -> Divide/2
  TxReq/1 -> Chart/1(TxReq)
  Divide/1 -> Data Type Conversion/1
  Chart/1(TxTrigger()) -> TxTrigger/1
  Gain/1 -> Divide/1
  Constant3/1 -> Gain/1
  Data Type Conversion/1 -> Chart/2(CycleCnt)

== system halout/HAL_OUT/CAN4/FD4_C100_0_0xCF103D0 ==
  BSCP_outputs : Inport  OutDataTypeStr=Bus: BSCP_outputs
  BOUTP_outputs : Inport  Port=2  OutDataTypeStr=Bus: BOUTP_outputs
  DCDCEnDemand : Subsystem
  EACSpdDemand : Subsystem
  FDCCHAEACEnDemandCmd : Subsystem
  FDCEHPSEnDemandCmd : Subsystem
  FDCEHPSSpdDemandCmd : Subsystem
  VCULife2 : Subsystem
  bus_creator : BusCreator  Inputs=6  OutDataTypeStr=Bus: DT_CAN4_SG_FD4_C100_0  NonVirtualBus=on
  bus_selector : BusSelector  OutputSignals=VOUTP_DCDCEnDemamd_enum
  bus_selector1 : BusSelector  OutputSignals=VOUTP_EACSpdDemand_rpm
  bus_selector2 : BusSelector  OutputSignals=VOUTP_EACEnDemand_enum
  bus_selector3 : BusSelector  OutputSignals=VOUTP_EHPSEnDemand_enum
  bus_selector4 : BusSelector  OutputSignals=VOUTP_EHPSMotorDemSpd_rpm
  bus_selector5 : BusSelector  OutputSignals=VOUTP_VCULife2_cnt
  FD4_C100_0 : Outport
  wires:
  BSCP_outputs/1 -> [BSCP_outputs]
  BOUTP_outputs/1 -> [BOUTP_outputs]
  [CAN4_DCDCEnDemand] -> bus_creator/1  "CAN4_DCDCEnDemand"
  [CAN4_EACSpdDemand] -> bus_creator/2  "CAN4_EACSpdDemand"
  [CAN4_FDC_CHA_EACEnDemand_Cmd] -> bus_creator/3  "CAN4_FDC_CHA_EACEnDemand_Cmd"
  [CAN4_FDC_EHPS_EnDemand_Cmd] -> bus_creator/4  "CAN4_FDC_EHPS_EnDemand_Cmd"
  [CAN4_FDC_EHPS_SpdDemand_Cmd] -> bus_creator/5  "CAN4_FDC_EHPS_SpdDemand_Cmd"
  [CAN4_VCULife2] -> bus_creator/6  "CAN4_VCULife2"
  bus_creator/1 -> FD4_C100_0/1
  DCDCEnDemand/1(CAN4_DCDCEnDemand) -> [CAN4_DCDCEnDemand]
  EACSpdDemand/1(CAN4_EACSpdDemand) -> [CAN4_EACSpdDemand]
  FDCCHAEACEnDemandCmd/1(CAN4_FDC_CHA_EACEnDemand_Cmd) -> [CAN4_FDC_CHA_EACEnDemand_Cmd]
  FDCEHPSEnDemandCmd/1(CAN4_FDC_EHPS_EnDemand_Cmd) -> [CAN4_FDC_EHPS_EnDemand_Cmd]
  FDCEHPSSpdDemandCmd/1(CAN4_FDC_EHPS_SpdDemand_Cmd) -> [CAN4_FDC_EHPS_SpdDemand_Cmd]
  VCULife2/1(CAN4_VCULife2) -> [CAN4_VCULife2]
  bus_selector/1 -> DCDCEnDemand/1(DCDCEnDemand)  "<VOUTP_DCDCEnDemamd_enum>"
  [BOUTP_outputs] -> bus_selector/1
  bus_selector1/1 -> EACSpdDemand/1(EACSpdDemand)  "<VOUTP_EACSpdDemand_rpm>"
  [BOUTP_outputs] -> bus_selector1/1
  bus_selector2/1 -> FDCCHAEACEnDemandCmd/1(FDCCHAEACEnDemandCmd)  "<VOUTP_EACEnDemand_enum>"
  [BOUTP_outputs] -> bus_selector2/1
  bus_selector3/1 -> FDCEHPSEnDemandCmd/1(FDCEHPSEnDemandCmd)  "<VOUTP_EHPSEnDemand_enum>"
  [BOUTP_outputs] -> bus_selector3/1
  bus_selector4/1 -> FDCEHPSSpdDemandCmd/1(FDCEHPSSpdDemandCmd)  "<VOUTP_EHPSMotorDemSpd_rpm>"
  [BOUTP_outputs] -> bus_selector4/1
  bus_selector5/1 -> VCULife2/1(VCULife2)  "<VOUTP_VCULife2_cnt>"
  [BOUTP_outputs] -> bus_selector5/1

== system halout/HAL_OUT/CAN4/FD4_C10_0_0xCF101D0 ==
  BSCP_outputs : Inport  OutDataTypeStr=Bus: BSCP_outputs
  BOUTP_outputs : Inport  Port=2  OutDataTypeStr=Bus: BOUTP_outputs
  ACHVPwrOnOffReq : Subsystem
  MCUHVPwrOnOffReq : Subsystem
  VCUDCDCEACEHPSRlyEncmd : Subsystem
  VCUDeFogTMSRlyEncmd : Subsystem
  VCULife1 : Subsystem
  bus_creator : BusCreator  Inputs=5  OutDataTypeStr=Bus: DT_CAN4_SG_FD4_C10_0  NonVirtualBus=on
  bus_selector : BusSelector  OutputSignals=VOUTP_ACHVLoopDem_enum
  bus_selector1 : BusSelector  OutputSignals=VOUTP_MCUHVLoopDem_enum
  bus_selector2 : BusSelector  OutputSignals=VOUTP_VCULife1_cnt
  bus_selector3 : BusSelector  OutputSignals=VOUTP_DCDCRlyDem_enum
  bus_selector4 : BusSelector  OutputSignals=VOUTP_FogTMSRlyCMD_enum
  FD4_C10_0 : Outport
  wires:
  BSCP_outputs/1 -> [BSCP_outputs]
  BOUTP_outputs/1 -> [BOUTP_outputs]
  [CAN4_ACHVPwrOnOffReq] -> bus_creator/1  "CAN4_ACHVPwrOnOffReq"
  [CAN4_MCUHVPwrOnOffReq] -> bus_creator/2  "CAN4_MCUHVPwrOnOffReq"
  [CAN4_VCULife1] -> bus_creator/3  "CAN4_VCULife1"
  [CAN4_VCU_DCDCEACEHPSRlyEn_cmd] -> bus_creator/4  "CAN4_VCU_DCDCEACEHPSRlyEn_cmd"
  [CAN4_VCU_DeFogTMSRlyEn_cmd] -> bus_creator/5  "CAN4_VCU_DeFogTMSRlyEn_cmd"
  bus_creator/1 -> FD4_C10_0/1
  ACHVPwrOnOffReq/1(CAN4_ACHVPwrOnOffReq) -> [CAN4_ACHVPwrOnOffReq]
  MCUHVPwrOnOffReq/1(CAN4_MCUHVPwrOnOffReq) -> [CAN4_MCUHVPwrOnOffReq]
  VCULife1/1(CAN4_VCULife1) -> [CAN4_VCULife1]
  VCUDCDCEACEHPSRlyEncmd/1(CAN4_VCU_DCDCEACEHPSRlyEn_cmd) -> [CAN4_VCU_DCDCEACEHPSRlyEn_cmd]
  VCUDeFogTMSRlyEncmd/1(CAN4_VCU_DeFogTMSRlyEn_cmd) -> [CAN4_VCU_DeFogTMSRlyEn_cmd]
  bus_selector/1 -> ACHVPwrOnOffReq/1(ACHVPwrOnOffReq)  "<VOUTP_ACHVLoopDem_enum>"
  [BOUTP_outputs] -> bus_selector/1
  bus_selector1/1 -> MCUHVPwrOnOffReq/1(MCUHVPwrOnOffReq)  "<VOUTP_MCUHVLoopDem_enum>"
  [BOUTP_outputs] -> bus_selector1/1
  bus_selector2/1 -> VCULife1/1(VCULife1)  "<VOUTP_VCULife1_cnt>"
  [BOUTP_outputs] -> bus_selector2/1
  bus_selector3/1 -> VCUDCDCEACEHPSRlyEncmd/1(VCUDCDCEACEHPSRlyEncmd)  "<VOUTP_DCDCRlyDem_enum>"
  [BOUTP_outputs] -> bus_selector3/1
  bus_selector4/1 -> VCUDeFogTMSRlyEncmd/1(VCUDeFogTMSRlyEncmd)  "<VOUTP_FogTMSRlyCMD_enum>"
  [BOUTP_outputs] -> bus_selector4/1

== system halout/HAL_OUT/CAN4/FD4_C200_0_0x18F003EF ==
  BSCP_outputs : Inport  OutDataTypeStr=Bus: BSCP_outputs
  BOUTP_outputs : Inport  Port=2  OutDataTypeStr=Bus: BOUTP_outputs
  SysPowerMode : Subsystem
  VCUIGNSta : Subsystem
  VCUIRCSta : Subsystem
  bus_creator : BusCreator  Inputs=3  OutDataTypeStr=Bus: DT_CAN4_SG_FD4_C200_0  NonVirtualBus=on
  bus_selector : BusSelector  OutputSignals=VOUTP_SysPowerMode_enum
  bus_selector1 : BusSelector  OutputSignals=VOUTP_IGNRlyClose_flg
  bus_selector2 : BusSelector  OutputSignals=VOUTP_IRCRlyClose_flg
  FD4_C200_0 : Outport
  wires:
  BSCP_outputs/1 -> [BSCP_outputs]
  BOUTP_outputs/1 -> [BOUTP_outputs]
  [CAN4_SysPowerMode] -> bus_creator/1  "CAN4_SysPowerMode"
  [CAN4_VCUIGNSta] -> bus_creator/2  "CAN4_VCUIGNSta"
  [CAN4_VCUIRCSta] -> bus_creator/3  "CAN4_VCUIRCSta"
  bus_creator/1 -> FD4_C200_0/1
  SysPowerMode/1(CAN4_SysPowerMode) -> [CAN4_SysPowerMode]
  VCUIGNSta/1(CAN4_VCUIGNSta) -> [CAN4_VCUIGNSta]
  VCUIRCSta/1(CAN4_VCUIRCSta) -> [CAN4_VCUIRCSta]
  bus_selector/1 -> SysPowerMode/1(SysPowerMode)  "<VOUTP_SysPowerMode_enum>"
  [BOUTP_outputs] -> bus_selector/1
  bus_selector1/1 -> VCUIGNSta/1(VCUIGNSta)  "<VOUTP_IGNRlyClose_flg>"
  [BOUTP_outputs] -> bus_selector1/1
  bus_selector2/1 -> VCUIRCSta/1(VCUIRCSta)  "<VOUTP_IRCRlyClose_flg>"
  [BOUTP_outputs] -> bus_selector2/1

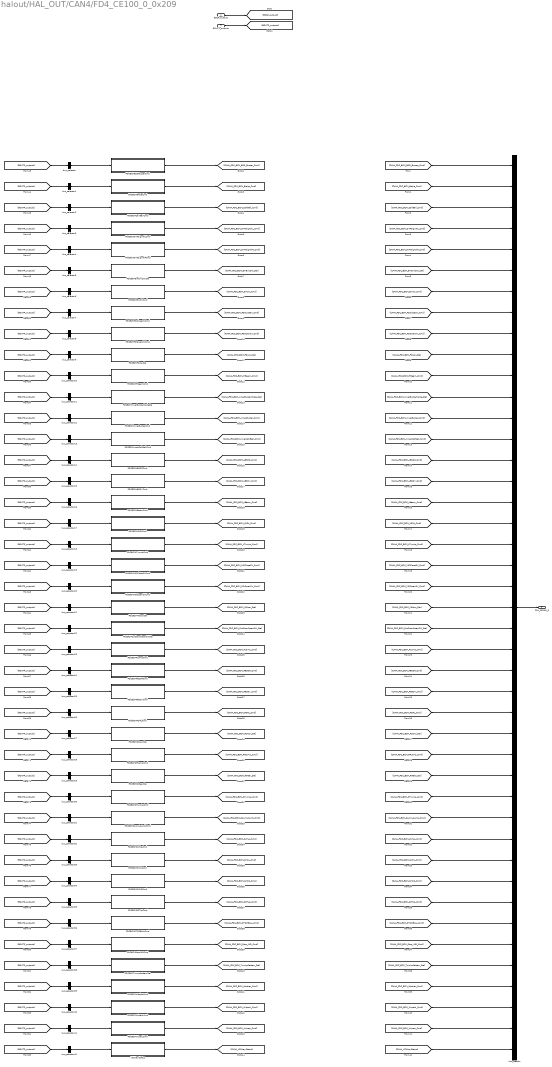
== system halout/HAL_OUT/CAN4/FD4_CE100_0_0x209 ==
  BSCP_outputs : Inport  OutDataTypeStr=Bus: BSCP_outputs
  BOUTP_outputs : Inport  Port=2  OutDataTypeStr=Bus: BOUTP_outputs
  FDCBCMBSDBuzzerCmd : Subsystem
  FDCBCMBrakeCmd : Subsystem
  FDCBCMCallBellCmd : Subsystem
  FDCBCMDVRSignalLCmd : Subsystem
  FDCBCMDVRSignalRCmd : Subsystem
  FDCBCMEmExitSWSta : Subsystem
  FDCBCMEmSVCmd : Subsystem
  FDCBCMFDCloseSVCmd : Subsystem
  FDCBCMFDOpenSVCmd : Subsystem
  FDCBCMFDoorSta : Subsystem
  FDCBCMHBeamCmd : Subsystem
  FDCBCMInnerBuzzerCmd : Subsystem
  FDCBCMInnerBuzzerModeSta : Subsystem
  FDCBCMInnerCallBellCmd : Subsystem
  FDCBCMLBSDRCmd : Subsystem
  FDCBCMLBSDYCmd : Subsystem
  FDCBCMLBeamCmd : Subsystem
  FDCBCMLDRLCmd : Subsystem
  FDCBCMLTurnLpCmd : Subsystem
  FDCBCMMDCloseSVCmd : Subsystem
  FDCBCMMDOpenSVCmd : Subsystem
  FDCBCMMDoorSta : Subsystem
  FDCBCMOutDoorOpenSWSta : Subsystem
  FDCBCMPLampCmd : Subsystem
  FDCBCMRBSDRCmd : Subsystem
  FDCBCMRBSDYCmd : Subsystem
  FDCBCMRDRLCmd : Subsystem
  FDCBCMRDoorSta : Subsystem
  FDCBCMRFLampCmd : Subsystem
  FDCBCMRGearSta : Subsystem
  FDCBCMRTurnLpCmd : Subsystem
  FDCBCMRoomLpAmbCmd : Subsystem
  FDCBCMSLTLpCmd : Subsystem
  FDCBCMSMKLCmd : Subsystem
  FDCBCMSMKRCmd : Subsystem
  FDCBCMSRTLpCmd : Subsystem
  FDCBCMSTOPBALLCmd : Subsystem
  FDCBCMStopINDCmd : Subsystem
  FDCBCMTurnLpPatternSta : Subsystem
  FDCBCMWasherCmd : Subsystem
  FDCBCMWiperHCmd : Subsystem
  FDCBCMWiperLCmd : Subsystem
  VCUKeyStatus : Subsystem
  bus_creator : BusCreator  Inputs=43  OutDataTypeStr=Bus: DT_CAN4_SG_FD4_CE100_0  NonVirtualBus=on
  bus_selector : BusSelector  OutputSignals=VOUTP_FDCBCMBSDBuzzerCmd_flg
  bus_selector1 : BusSelector  OutputSignals=VOUTP_FDCBCMBrakeCmd_flg
  bus_selector10 : BusSelector  OutputSignals=VOUTP_FDCBCMHBeamCmd_flg
  bus_selector11 : BusSelector  OutputSignals=VOUTP_InnerBuzzerModeSta_enum
  bus_selector12 : BusSelector  OutputSignals=VOUTP_FDCBCMInnerBuzzerCmd_flg
  bus_selector13 : BusSelector  OutputSignals=VOUTP_FDCBCMInnerCallBellCmd_flg
  bus_selector14 : BusSelector  OutputSignals=VOUTP_FDCBCMLBSDRCmd_flg
  bus_selector15 : BusSelector  OutputSignals=VOUTP_FDCBCMLBSDYCmd_flg
  bus_selector16 : BusSelector  OutputSignals=VOUTP_FDCBCMLBeamCmd_flg
  bus_selector17 : BusSelector  OutputSignals=VOUTP_FDCBCMLDRLCmd_flg
  bus_selector18 : BusSelector  OutputSignals=VOUTP_FDCBCMLTurnLpCmd_flg
  bus_selector19 : BusSelector  OutputSignals=VOUTP_FDCBCMMDCloseSVCmd_flg
  bus_selector2 : BusSelector  OutputSignals=VOUTP_FDCBCMCallBellCmd_flg
  bus_selector20 : BusSelector  OutputSignals=VOUTP_FDCBCMMDOpenSVCmd_flg
  bus_selector21 : BusSelector  OutputSignals=VOUTP_FDCBCMMDoorSta_flg
  bus_selector22 : BusSelector  OutputSignals=VOUTP_FDCBCMOSDrOpenSWSta_enum
  bus_selector23 : BusSelector  OutputSignals=VOUTP_FDCBCMPLampCmd_flg
  bus_selector24 : BusSelector  OutputSignals=VOUTP_FDCBCMRBSDRCmd_flg
  bus_selector25 : BusSelector  OutputSignals=VOUTP_FDCBCMRBSDYCmd_flg
  bus_selector26 : BusSelector  OutputSignals=VOUTP_FDCBCMRDRLCmd_flg
  bus_selector27 : BusSelector  OutputSignals=VOUTP_FDCBCMRDoorSta_flg
  bus_selector28 : BusSelector  OutputSignals=VOUTP_FDCBCMRFLampCmd_flg
  bus_selector29 : BusSelector  OutputSignals=VOUTP_FDCBCMRGearSta_flg
  bus_selector3 : BusSelector  OutputSignals=VOUTP_FDCBCMDVRSignalLCmd_flg
  bus_selector30 : BusSelector  OutputSignals=VOUTP_FDCBCMRTurnLpCmd_flg
  bus_selector31 : BusSelector  OutputSignals=VOUTP_FDCBCMRoomLpAmbCmd_flg
  bus_selector32 : BusSelector  OutputSignals=VOUTP_FDCBCMSLTLpCmd_flg
  bus_selector33 : BusSelector  OutputSignals=VOUTP_FDCBCMSMKLCmd_flg
  bus_selector34 : BusSelector  OutputSignals=VOUTP_FDCBCMSMKRCmd_flg
  bus_selector35 : BusSelector  OutputSignals=VOUTP_FDCBCMSRTLpCmd_flg
  bus_selector36 : BusSelector  OutputSignals=VOUTP_FDCBCMSTOPBALLCmd_flg
  bus_selector37 : BusSelector  OutputSignals=VOUTP_FDCBCMStopINDCmd_flg
  bus_selector38 : BusSelector  OutputSignals=VOUTP_TurnLpPatternSta_enum
  bus_selector39 : BusSelector  OutputSignals=VOUTP_FDCBCMWasherCmd_flg
  bus_selector4 : BusSelector  OutputSignals=VOUTP_FDCBCMDVRSignalRCmd_flg
  bus_selector40 : BusSelector  OutputSignals=VOUTP_FDCBCMWiperHCmd_flg
  bus_selector41 : BusSelector  OutputSignals=VOUTP_FDCBCMWiperLCmd_flg
  bus_selector42 : BusSelector  OutputSignals=VOUTP_Keystatus_enum
  bus_selector5 : BusSelector  OutputSignals=VOUTP_FDCBCMEmExitSWSta_flg
  bus_selector6 : BusSelector  OutputSignals=VOUTP_FDCBCMEmSVCmd_flg
  bus_selector7 : BusSelector  OutputSignals=VOUTP_FDCBCMFDCloseSVCmd_flg
  bus_selector8 : BusSelector  OutputSignals=VOUTP_FDCBCMFDOpenSVCmd_flg
  bus_selector9 : BusSelector  OutputSignals=VOUTP_FDCBCMFDoorSta_flg
  FD4_CE100_0 : Outport
  wires:
  BSCP_outputs/1 -> [BSCP_outputs]
  BOUTP_outputs/1 -> [BOUTP_outputs]
  [CAN4_FDC_BCM_BSD_Buzzer_Cmd] -> bus_creator/1  "CAN4_FDC_BCM_BSD_Buzzer_Cmd"
  [CAN4_FDC_BCM_Brake_Cmd] -> bus_creator/2  "CAN4_FDC_BCM_Brake_Cmd"
  [CAN4_FDC_BCM_CallBell_Cmd] -> bus_creator/3  "CAN4_FDC_BCM_CallBell_Cmd"
  [CAN4_FDC_BCM_DVRSignalL_Cmd] -> bus_creator/4  "CAN4_FDC_BCM_DVRSignalL_Cmd"
  [CAN4_FDC_BCM_DVRSignalR_Cmd] -> bus_creator/5  "CAN4_FDC_BCM_DVRSignalR_Cmd"
  [CAN4_FDC_BCM_EmExitSW_Sta] -> bus_creator/6  "CAN4_FDC_BCM_EmExitSW_Sta"
  [CAN4_FDC_BCM_EmSV_Cmd] -> bus_creator/7  "CAN4_FDC_BCM_EmSV_Cmd"
  [CAN4_FDC_BCM_FDCloseSV_Cmd] -> bus_creator/8  "CAN4_FDC_BCM_FDCloseSV_Cmd"
  [CAN4_FDC_BCM_FDOpenSV_Cmd] -> bus_creator/9  "CAN4_FDC_BCM_FDOpenSV_Cmd"
  [CAN4_FDC_BCM_FDoor_Sta] -> bus_creator/10  "CAN4_FDC_BCM_FDoor_Sta"
  [CAN4_FDC_BCM_HBeam_Cmd] -> bus_creator/11  "CAN4_FDC_BCM_HBeam_Cmd"
  [CAN4_FDC_BCM_InnerBuzzerMode_Sta] -> bus_creator/12  "CAN4_FDC_BCM_InnerBuzzerMode_Sta"
  [CAN4_FDC_BCM_InnerBuzzer_Cmd] -> bus_creator/13  "CAN4_FDC_BCM_InnerBuzzer_Cmd"
  [CAN4_FDC_BCM_InnerCallBell_Cmd] -> bus_creator/14  "CAN4_FDC_BCM_InnerCallBell_Cmd"
  [CAN4_FDC_BCM_LBSDR_Cmd] -> bus_creator/15  "CAN4_FDC_BCM_LBSDR_Cmd"
  [CAN4_FDC_BCM_LBSDY_Cmd] -> bus_creator/16  "CAN4_FDC_BCM_LBSDY_Cmd"
  [CAN4_FDC_BCM_LBeam_Cmd] -> bus_creator/17  "CAN4_FDC_BCM_LBeam_Cmd"
  [CAN4_FDC_BCM_LDRL_Cmd] -> bus_creator/18  "CAN4_FDC_BCM_LDRL_Cmd"
  [CAN4_FDC_BCM_LTurnLp_Cmd] -> bus_creator/19  "CAN4_FDC_BCM_LTurnLp_Cmd"
  [CAN4_FDC_BCM_MDCloseSV_Cmd] -> bus_creator/20  "CAN4_FDC_BCM_MDCloseSV_Cmd"
  [CAN4_FDC_BCM_MDOpenSV_Cmd] -> bus_creator/21  "CAN4_FDC_BCM_MDOpenSV_Cmd"
  [CAN4_FDC_BCM_MDoor_Sta] -> bus_creator/22  "CAN4_FDC_BCM_MDoor_Sta"
  [CAN4_FDC_BCM_OutDoorOpenSW_Sta] -> bus_creator/23  "CAN4_FDC_BCM_OutDoorOpenSW_Sta"
  [CAN4_FDC_BCM_PLamp_Cmd] -> bus_creator/24  "CAN4_FDC_BCM_PLamp_Cmd"
  [CAN4_FDC_BCM_RBSDR_Cmd] -> bus_creator/25  "CAN4_FDC_BCM_RBSDR_Cmd"
  [CAN4_FDC_BCM_RBSDY_Cmd] -> bus_creator/26  "CAN4_FDC_BCM_RBSDY_Cmd"
  [CAN4_FDC_BCM_RDRL_Cmd] -> bus_creator/27  "CAN4_FDC_BCM_RDRL_Cmd"
  [CAN4_FDC_BCM_RDoor_Sta] -> bus_creator/28  "CAN4_FDC_BCM_RDoor_Sta"
  [CAN4_FDC_BCM_RFLamp_Cmd] -> bus_creator/29  "CAN4_FDC_BCM_RFLamp_Cmd"
  [CAN4_FDC_BCM_RGear_Sta] -> bus_creator/30  "CAN4_FDC_BCM_RGear_Sta"
  [CAN4_FDC_BCM_RTurnLp_Cmd] -> bus_creator/31  "CAN4_FDC_BCM_RTurnLp_Cmd"
  [CAN4_FDC_BCM_RoomLpAmb_Cmd] -> bus_creator/32  "CAN4_FDC_BCM_RoomLpAmb_Cmd"
  [CAN4_FDC_BCM_SLTLp_Cmd] -> bus_creator/33  "CAN4_FDC_BCM_SLTLp_Cmd"
  [CAN4_FDC_BCM_SMKL_Cmd] -> bus_creator/34  "CAN4_FDC_BCM_SMKL_Cmd"
  [CAN4_FDC_BCM_SMKR_Cmd] -> bus_creator/35  "CAN4_FDC_BCM_SMKR_Cmd"
  [CAN4_FDC_BCM_SRTLp_Cmd] -> bus_creator/36  "CAN4_FDC_BCM_SRTLp_Cmd"
  [CAN4_FDC_BCM_STOPBALL_Cmd] -> bus_creator/37  "CAN4_FDC_BCM_STOPBALL_Cmd"
  [CAN4_FDC_BCM_Stop_IND_Cmd] -> bus_creator/38  "CAN4_FDC_BCM_Stop_IND_Cmd"
  [CAN4_FDC_BCM_TurnLpPattern_Sta] -> bus_creator/39  "CAN4_FDC_BCM_TurnLpPattern_Sta"
  [CAN4_FDC_BCM_Washer_Cmd] -> bus_creator/40  "CAN4_FDC_BCM_Washer_Cmd"
  [CAN4_FDC_BCM_WiperH_Cmd] -> bus_creator/41  "CAN4_FDC_BCM_WiperH_Cmd"
  [CAN4_FDC_BCM_WiperL_Cmd] -> bus_creator/42  "CAN4_FDC_BCM_WiperL_Cmd"
  [CAN4_VCUKeyStatus] -> bus_creator/43  "CAN4_VCUKeyStatus"
  bus_creator/1 -> FD4_CE100_0/1
  FDCBCMBSDBuzzerCmd/1(CAN4_FDC_BCM_BSD_Buzzer_Cmd) -> [CAN4_FDC_BCM_BSD_Buzzer_Cmd]
  FDCBCMBrakeCmd/1(CAN4_FDC_BCM_Brake_Cmd) -> [CAN4_FDC_BCM_Brake_Cmd]
  FDCBCMCallBellCmd/1(CAN4_FDC_BCM_CallBell_Cmd) -> [CAN4_FDC_BCM_CallBell_Cmd]
  FDCBCMDVRSignalLCmd/1(CAN4_FDC_BCM_DVRSignalL_Cmd) -> [CAN4_FDC_BCM_DVRSignalL_Cmd]
  FDCBCMDVRSignalRCmd/1(CAN4_FDC_BCM_DVRSignalR_Cmd) -> [CAN4_FDC_BCM_DVRSignalR_Cmd]
  FDCBCMEmExitSWSta/1(CAN4_FDC_BCM_EmExitSW_Sta) -> [CAN4_FDC_BCM_EmExitSW_Sta]
  FDCBCMEmSVCmd/1(CAN4_FDC_BCM_EmSV_Cmd) -> [CAN4_FDC_BCM_EmSV_Cmd]
  FDCBCMFDCloseSVCmd/1(CAN4_FDC_BCM_FDCloseSV_Cmd) -> [CAN4_FDC_BCM_FDCloseSV_Cmd]
  FDCBCMFDOpenSVCmd/1(CAN4_FDC_BCM_FDOpenSV_Cmd) -> [CAN4_FDC_BCM_FDOpenSV_Cmd]
  FDCBCMFDoorSta/1(CAN4_FDC_BCM_FDoor_Sta) -> [CAN4_FDC_BCM_FDoor_Sta]
  FDCBCMHBeamCmd/1(CAN4_FDC_BCM_HBeam_Cmd) -> [CAN4_FDC_BCM_HBeam_Cmd]
  FDCBCMInnerBuzzerModeSta/1(CAN4_FDC_BCM_InnerBuzzerMode_Sta) -> [CAN4_FDC_BCM_InnerBuzzerMode_Sta]
  FDCBCMInnerBuzzerCmd/1(CAN4_FDC_BCM_InnerBuzzer_Cmd) -> [CAN4_FDC_BCM_InnerBuzzer_Cmd]
  FDCBCMInnerCallBellCmd/1(CAN4_FDC_BCM_InnerCallBell_Cmd) -> [CAN4_FDC_BCM_InnerCallBell_Cmd]
  FDCBCMLBSDRCmd/1(CAN4_FDC_BCM_LBSDR_Cmd) -> [CAN4_FDC_BCM_LBSDR_Cmd]
  FDCBCMLBSDYCmd/1(CAN4_FDC_BCM_LBSDY_Cmd) -> [CAN4_FDC_BCM_LBSDY_Cmd]
  FDCBCMLBeamCmd/1(CAN4_FDC_BCM_LBeam_Cmd) -> [CAN4_FDC_BCM_LBeam_Cmd]
  FDCBCMLDRLCmd/1(CAN4_FDC_BCM_LDRL_Cmd) -> [CAN4_FDC_BCM_LDRL_Cmd]
  FDCBCMLTurnLpCmd/1(CAN4_FDC_BCM_LTurnLp_Cmd) -> [CAN4_FDC_BCM_LTurnLp_Cmd]
  FDCBCMMDCloseSVCmd/1(CAN4_FDC_BCM_MDCloseSV_Cmd) -> [CAN4_FDC_BCM_MDCloseSV_Cmd]
  FDCBCMMDOpenSVCmd/1(CAN4_FDC_BCM_MDOpenSV_Cmd) -> [CAN4_FDC_BCM_MDOpenSV_Cmd]
  FDCBCMMDoorSta/1(CAN4_FDC_BCM_MDoor_Sta) -> [CAN4_FDC_BCM_MDoor_Sta]
  FDCBCMOutDoorOpenSWSta/1(CAN4_FDC_BCM_OutDoorOpenSW_Sta) -> [CAN4_FDC_BCM_OutDoorOpenSW_Sta]
  FDCBCMPLampCmd/1(CAN4_FDC_BCM_PLamp_Cmd) -> [CAN4_FDC_BCM_PLamp_Cmd]
  FDCBCMRBSDRCmd/1(CAN4_FDC_BCM_RBSDR_Cmd) -> [CAN4_FDC_BCM_RBSDR_Cmd]
  FDCBCMRBSDYCmd/1(CAN4_FDC_BCM_RBSDY_Cmd) -> [CAN4_FDC_BCM_RBSDY_Cmd]
  FDCBCMRDRLCmd/1(CAN4_FDC_BCM_RDRL_Cmd) -> [CAN4_FDC_BCM_RDRL_Cmd]
  FDCBCMRDoorSta/1(CAN4_FDC_BCM_RDoor_Sta) -> [CAN4_FDC_BCM_RDoor_Sta]
  FDCBCMRFLampCmd/1(CAN4_FDC_BCM_RFLamp_Cmd) -> [CAN4_FDC_BCM_RFLamp_Cmd]
  FDCBCMRGearSta/1(CAN4_FDC_BCM_RGear_Sta) -> [CAN4_FDC_BCM_RGear_Sta]
  FDCBCMRTurnLpCmd/1(CAN4_FDC_BCM_RTurnLp_Cmd) -> [CAN4_FDC_BCM_RTurnLp_Cmd]
  FDCBCMRoomLpAmbCmd/1(CAN4_FDC_BCM_RoomLpAmb_Cmd) -> [CAN4_FDC_BCM_RoomLpAmb_Cmd]
  FDCBCMSLTLpCmd/1(CAN4_FDC_BCM_SLTLp_Cmd) -> [CAN4_FDC_BCM_SLTLp_Cmd]
  FDCBCMSMKLCmd/1(CAN4_FDC_BCM_SMKL_Cmd) -> [CAN4_FDC_BCM_SMKL_Cmd]
  FDCBCMSMKRCmd/1(CAN4_FDC_BCM_SMKR_Cmd) -> [CAN4_FDC_BCM_SMKR_Cmd]
  FDCBCMSRTLpCmd/1(CAN4_FDC_BCM_SRTLp_Cmd) -> [CAN4_FDC_BCM_SRTLp_Cmd]
  FDCBCMSTOPBALLCmd/1(CAN4_FDC_BCM_STOPBALL_Cmd) -> [CAN4_FDC_BCM_STOPBALL_Cmd]
  FDCBCMStopINDCmd/1(CAN4_FDC_BCM_Stop_IND_Cmd) -> [CAN4_FDC_BCM_Stop_IND_Cmd]
  FDCBCMTurnLpPatternSta/1(CAN4_FDC_BCM_TurnLpPattern_Sta) -> [CAN4_FDC_BCM_TurnLpPattern_Sta]
  FDCBCMWasherCmd/1(CAN4_FDC_BCM_Washer_Cmd) -> [CAN4_FDC_BCM_Washer_Cmd]
  FDCBCMWiperHCmd/1(CAN4_FDC_BCM_WiperH_Cmd) -> [CAN4_FDC_BCM_WiperH_Cmd]
  FDCBCMWiperLCmd/1(CAN4_FDC_BCM_WiperL_Cmd) -> [CAN4_FDC_BCM_WiperL_Cmd]
  VCUKeyStatus/1(CAN4_VCUKeyStatus) -> [CAN4_VCUKeyStatus]
  bus_selector/1 -> FDCBCMBSDBuzzerCmd/1(FDCBCMBSDBuzzerCmd)  "<VOUTP_FDCBCMBSDBuzzerCmd_flg>"
  [BOUTP_outputs] -> bus_selector/1
  bus_selector1/1 -> FDCBCMBrakeCmd/1(FDCBCMBrakeCmd)  "<VOUTP_FDCBCMBrakeCmd_flg>"
  [BOUTP_outputs] -> bus_selector1/1
  bus_selector2/1 -> FDCBCMCallBellCmd/1(FDCBCMCallBellCmd)  "<VOUTP_FDCBCMCallBellCmd_flg>"
  [BOUTP_outputs] -> bus_selector2/1
  bus_selector3/1 -> FDCBCMDVRSignalLCmd/1(FDCBCMDVRSignalLCmd)  "<VOUTP_FDCBCMDVRSignalLCmd_flg>"
  [BOUTP_outputs] -> bus_selector3/1
  bus_selector4/1 -> FDCBCMDVRSignalRCmd/1(FDCBCMDVRSignalRCmd)  "<VOUTP_FDCBCMDVRSignalRCmd_flg>"
  [BOUTP_outputs] -> bus_selector4/1
  bus_selector5/1 -> FDCBCMEmExitSWSta/1(FDCBCMEmExitSWSta)  "<VOUTP_FDCBCMEmExitSWSta_flg>"
  [BOUTP_outputs] -> bus_selector5/1
  bus_selector6/1 -> FDCBCMEmSVCmd/1(FDCBCMEmSVCmd)  "<VOUTP_FDCBCMEmSVCmd_flg>"
  [BOUTP_outputs] -> bus_selector6/1
  bus_selector7/1 -> FDCBCMFDCloseSVCmd/1(FDCBCMFDCloseSVCmd)  "<VOUTP_FDCBCMFDCloseSVCmd_flg>"
  [BOUTP_outputs] -> bus_selector7/1
  bus_selector8/1 -> FDCBCMFDOpenSVCmd/1(FDCBCMFDOpenSVCmd)  "<VOUTP_FDCBCMFDOpenSVCmd_flg>"
  [BOUTP_outputs] -> bus_selector8/1
  bus_selector9/1 -> FDCBCMFDoorSta/1(FDCBCMFDoorSta)  "<VOUTP_FDCBCMFDoorSta_flg>"
  [BOUTP_outputs] -> bus_selector9/1
  bus_selector10/1 -> FDCBCMHBeamCmd/1(FDCBCMHBeamCmd)  "<VOUTP_FDCBCMHBeamCmd_flg>"
  [BOUTP_outputs] -> bus_selector10/1
  bus_selector11/1 -> FDCBCMInnerBuzzerModeSta/1(FDCBCMInnerBuzzerModeSta)  "<VOUTP_InnerBuzzerModeSta_enum>"
  [BOUTP_outputs] -> bus_selector11/1
  bus_selector12/1 -> FDCBCMInnerBuzzerCmd/1(FDCBCMInnerBuzzerCmd)  "<VOUTP_FDCBCMInnerBuzzerCmd_flg>"
  [BOUTP_outputs] -> bus_selector12/1
  bus_selector13/1 -> FDCBCMInnerCallBellCmd/1(FDCBCMInnerCallBellCmd)  "<VOUTP_FDCBCMInnerCallBellCmd_flg>"
  [BOUTP_outputs] -> bus_selector13/1
  bus_selector14/1 -> FDCBCMLBSDRCmd/1(FDCBCMLBSDRCmd)  "<VOUTP_FDCBCMLBSDRCmd_flg>"
  [BOUTP_outputs] -> bus_selector14/1
  bus_selector15/1 -> FDCBCMLBSDYCmd/1(FDCBCMLBSDYCmd)  "<VOUTP_FDCBCMLBSDYCmd_flg>"
  [BOUTP_outputs] -> bus_selector15/1
  bus_selector16/1 -> FDCBCMLBeamCmd/1(FDCBCMLBeamCmd)  "<VOUTP_FDCBCMLBeamCmd_flg>"
  [BOUTP_outputs] -> bus_selector16/1
  bus_selector17/1 -> FDCBCMLDRLCmd/1(FDCBCMLDRLCmd)  "<VOUTP_FDCBCMLDRLCmd_flg>"
  [BOUTP_outputs] -> bus_selector17/1
  bus_selector18/1 -> FDCBCMLTurnLpCmd/1(FDCBCMLTurnLpCmd)  "<VOUTP_FDCBCMLTurnLpCmd_flg>"
  [BOUTP_outputs] -> bus_selector18/1
  bus_selector19/1 -> FDCBCMMDCloseSVCmd/1(FDCBCMMDCloseSVCmd)  "<VOUTP_FDCBCMMDCloseSVCmd_flg>"
  [BOUTP_outputs] -> bus_selector19/1
  bus_selector20/1 -> FDCBCMMDOpenSVCmd/1(FDCBCMMDOpenSVCmd)  "<VOUTP_FDCBCMMDOpenSVCmd_flg>"
  [BOUTP_outputs] -> bus_selector20/1
  bus_selector21/1 -> FDCBCMMDoorSta/1(FDCBCMMDoorSta)  "<VOUTP_FDCBCMMDoorSta_flg>"
  [BOUTP_outputs] -> bus_selector21/1
  bus_selector22/1 -> FDCBCMOutDoorOpenSWSta/1(FDCBCMOutDoorOpenSWSta)  "<VOUTP_FDCBCMOSDrOpenSWSta_enum>"
  [BOUTP_outputs] -> bus_selector22/1
  bus_selector23/1 -> FDCBCMPLampCmd/1(FDCBCMPLampCmd)  "<VOUTP_FDCBCMPLampCmd_flg>"
  [BOUTP_outputs] -> bus_selector23/1
  bus_selector24/1 -> FDCBCMRBSDRCmd/1(FDCBCMRBSDRCmd)  "<VOUTP_FDCBCMRBSDRCmd_flg>"
  [BOUTP_outputs] -> bus_selector24/1
  bus_selector25/1 -> FDCBCMRBSDYCmd/1(FDCBCMRBSDYCmd)  "<VOUTP_FDCBCMRBSDYCmd_flg>"
  [BOUTP_outputs] -> bus_selector25/1
  bus_selector26/1 -> FDCBCMRDRLCmd/1(FDCBCMRDRLCmd)  "<VOUTP_FDCBCMRDRLCmd_flg>"
  [BOUTP_outputs] -> bus_selector26/1
  bus_selector27/1 -> FDCBCMRDoorSta/1(FDCBCMRDoorSta)  "<VOUTP_FDCBCMRDoorSta_flg>"
  [BOUTP_outputs] -> bus_selector27/1
  bus_selector28/1 -> FDCBCMRFLampCmd/1(FDCBCMRFLampCmd)  "<VOUTP_FDCBCMRFLampCmd_flg>"
  [BOUTP_outputs] -> bus_selector28/1
  bus_selector29/1 -> FDCBCMRGearSta/1(FDCBCMRGearSta)  "<VOUTP_FDCBCMRGearSta_flg>"
  [BOUTP_outputs] -> bus_selector29/1
  bus_selector30/1 -> FDCBCMRTurnLpCmd/1(FDCBCMRTurnLpCmd)  "<VOUTP_FDCBCMRTurnLpCmd_flg>"
  [BOUTP_outputs] -> bus_selector30/1
  bus_selector31/1 -> FDCBCMRoomLpAmbCmd/1(FDCBCMRoomLpAmbCmd)  "<VOUTP_FDCBCMRoomLpAmbCmd_flg>"
  [BOUTP_outputs] -> bus_selector31/1
  bus_selector32/1 -> FDCBCMSLTLpCmd/1(FDCBCMSLTLpCmd)  "<VOUTP_FDCBCMSLTLpCmd_flg>"
  [BOUTP_outputs] -> bus_selector32/1
  bus_selector33/1 -> FDCBCMSMKLCmd/1(FDCBCMSMKLCmd)  "<VOUTP_FDCBCMSMKLCmd_flg>"
  [BOUTP_outputs] -> bus_selector33/1
  bus_selector34/1 -> FDCBCMSMKRCmd/1(FDCBCMSMKRCmd)  "<VOUTP_FDCBCMSMKRCmd_flg>"
  [BOUTP_outputs] -> bus_selector34/1
  bus_selector35/1 -> FDCBCMSRTLpCmd/1(FDCBCMSRTLpCmd)  "<VOUTP_FDCBCMSRTLpCmd_flg>"
  [BOUTP_outputs] -> bus_selector35/1
  bus_selector36/1 -> FDCBCMSTOPBALLCmd/1(FDCBCMSTOPBALLCmd)  "<VOUTP_FDCBCMSTOPBALLCmd_flg>"
  [BOUTP_outputs] -> bus_selector36/1
  bus_selector37/1 -> FDCBCMStopINDCmd/1(FDCBCMStopINDCmd)  "<VOUTP_FDCBCMStopINDCmd_flg>"
  [BOUTP_outputs] -> bus_selector37/1
  bus_selector38/1 -> FDCBCMTurnLpPatternSta/1(FDCBCMTurnLpPatternSta)  "<VOUTP_TurnLpPatternSta_enum>"
  [BOUTP_outputs] -> bus_selector38/1
  bus_selector39/1 -> FDCBCMWasherCmd/1(FDCBCMWasherCmd)  "<VOUTP_FDCBCMWasherCmd_flg>"
  [BOUTP_outputs] -> bus_selector39/1
  bus_selector40/1 -> FDCBCMWiperHCmd/1(FDCBCMWiperHCmd)  "<VOUTP_FDCBCMWiperHCmd_flg>"
  [BOUTP_outputs] -> bus_selector40/1
  bus_selector41/1 -> FDCBCMWiperLCmd/1(FDCBCMWiperLCmd)  "<VOUTP_FDCBCMWiperLCmd_flg>"
  [BOUTP_outputs] -> bus_selector41/1
  bus_selector42/1 -> VCUKeyStatus/1(VCUKeyStatus)  "<VOUTP_Keystatus_enum>"
  [BOUTP_outputs] -> bus_selector42/1

== system halout/HAL_OUT/CAN4/FD4_CE100_1_0x210 ==
  BSCP_outputs : Inport  OutDataTypeStr=Bus: BSCP_outputs
  BOUTP_outputs : Inport  Port=2  OutDataTypeStr=Bus: BOUTP_outputs
  FDCBCMFRoomLpCmd : Subsystem
  FDCBCMMRoomLpCmd : Subsystem
  FDCBCMRRoomLpCmd : Subsystem
  FDCTHCMCoolFanReqCmd : Subsystem
  Ground : Ground
  Ground1 : Ground
  Ground2 : Ground
  bus_creator : BusCreator  Inputs=4  OutDataTypeStr=Bus: DT_CAN4_SG_FD4_CE100_1  NonVirtualBus=on
  bus_selector : BusSelector  OutputSignals=VOUTP_CoolFanReq_pct
  FD4_CE100_1 : Outport
  wires:
  BSCP_outputs/1 -> [BSCP_outputs]
  BOUTP_outputs/1 -> [BOUTP_outputs]
  [CAN4_FDC_BCM_FRoomLp_Cmd] -> bus_creator/1  "CAN4_FDC_BCM_FRoomLp_Cmd"
  [CAN4_FDC_BCM_MRoomLp_Cmd] -> bus_creator/2  "CAN4_FDC_BCM_MRoomLp_Cmd"
  [CAN4_FDC_BCM_RRoomLp_Cmd] -> bus_creator/3  "CAN4_FDC_BCM_RRoomLp_Cmd"
  [CAN4_FDC_THCM_CoolFanReq_Cmd] -> bus_creator/4  "CAN4_FDC_THCM_CoolFanReq_Cmd"
  bus_creator/1 -> FD4_CE100_1/1
  FDCBCMFRoomLpCmd/1(CAN4_FDC_BCM_FRoomLp_Cmd) -> [CAN4_FDC_BCM_FRoomLp_Cmd]
  FDCBCMMRoomLpCmd/1(CAN4_FDC_BCM_MRoomLp_Cmd) -> [CAN4_FDC_BCM_MRoomLp_Cmd]
  FDCBCMRRoomLpCmd/1(CAN4_FDC_BCM_RRoomLp_Cmd) -> [CAN4_FDC_BCM_RRoomLp_Cmd]
  FDCTHCMCoolFanReqCmd/1(CAN4_FDC_THCM_CoolFanReq_Cmd) -> [CAN4_FDC_THCM_CoolFanReq_Cmd]
  Ground/1 -> FDCBCMFRoomLpCmd/1(FDCBCMFRoomLpCmd)
  Ground1/1 -> FDCBCMMRoomLpCmd/1(FDCBCMMRoomLpCmd)
  Ground2/1 -> FDCBCMRRoomLpCmd/1(FDCBCMRRoomLpCmd)
  bus_selector/1 -> FDCTHCMCoolFanReqCmd/1(FDCTHCMCoolFanReqCmd)  "<VOUTP_CoolFanReq_pct>"
  [BOUTP_outputs] -> bus_selector/1

== system halout/HAL_OUT/CAN5/FD5_C100_0_0x18F348D0 ==
  BSCP_outputs : Inport  OutDataTypeStr=Bus: BSCP_outputs
  BOUTP_outputs : Inport  Port=2  OutDataTypeStr=Bus: BOUTP_outputs
  AlcLockSta : Subsystem
  B2VAPlusSta : Subsystem
  Ground : Ground
  Ground1 : Ground
  VCUHVILSta : Subsystem
  bus_creator : BusCreator  Inputs=3  OutDataTypeStr=Bus: DT_CAN5_SG_FD5_C100_0  NonVirtualBus=on
  bus_selector : BusSelector  OutputSignals=VOUTP_HVILFail_flg
  FD5_C100_0 : Outport
  wires:
  BSCP_outputs/1 -> [BSCP_outputs]
  BOUTP_outputs/1 -> [BOUTP_outputs]
  [CAN5_AlcLockSta] -> bus_creator/1  "CAN5_AlcLockSta"
  [CAN5_B2VAPlusSta] -> bus_creator/2  "CAN5_B2VAPlusSta"
  [CAN5_VCUHVILSta] -> bus_creator/3  "CAN5_VCUHVILSta"
  bus_creator/1 -> FD5_C100_0/1
  AlcLockSta/1(CAN5_AlcLockSta) -> [CAN5_AlcLockSta]
  B2VAPlusSta/1(CAN5_B2VAPlusSta) -> [CAN5_B2VAPlusSta]
  VCUHVILSta/1(CAN5_VCUHVILSta) -> [CAN5_VCUHVILSta]
  Ground/1 -> AlcLockSta/1(AlcLockSta)
  Ground1/1 -> B2VAPlusSta/1(B2VAPlusSta)
  bus_selector/1 -> VCUHVILSta/1(VCUHVILSta)  "<VOUTP_HVILFail_flg>"
  [BOUTP_outputs] -> bus_selector/1

== system halout/HAL_OUT/CAN5/FD5_C200_0_0x20D ==
  BSCP_outputs : Inport  OutDataTypeStr=Bus: BSCP_outputs
  BOUTP_outputs : Inport  Port=2  OutDataTypeStr=Bus: BOUTP_outputs
  SysPowerMode : Subsystem
  bus_creator : BusCreator  Inputs=1  OutDataTypeStr=Bus: DT_CAN5_SG_FD5_C200_0  NonVirtualBus=on
  bus_selector : BusSelector  OutputSignals=VOUTP_SysPowerMode_enum
  FD5_C200_0 : Outport
  wires:
  BSCP_outputs/1 -> [BSCP_outputs]
  BOUTP_outputs/1 -> [BOUTP_outputs]
  [CAN5_SysPowerMode] -> bus_creator/1  "CAN5_SysPowerMode"
  bus_creator/1 -> FD5_C200_0/1
  SysPowerMode/1(CAN5_SysPowerMode) -> [CAN5_SysPowerMode]
  bus_selector/1 -> SysPowerMode/1(SysPowerMode)  "<VOUTP_SysPowerMode_enum>"
  [BOUTP_outputs] -> bus_selector/1

== system halout/HAL_OUT/CAN6/FD6_C200_0_0x20C ==
  BSCP_outputs : Inport  OutDataTypeStr=Bus: BSCP_outputs
  BOUTP_outputs : Inport  Port=2  OutDataTypeStr=Bus: BOUTP_outputs
  SysPowerMode : Subsystem
  bus_creator : BusCreator  Inputs=1  OutDataTypeStr=Bus: DT_CAN6_SG_FD6_C200_0  NonVirtualBus=on
  bus_selector : BusSelector  OutputSignals=VOUTP_SysPowerMode_enum
  FD6_C200_0 : Outport
  wires:
  BSCP_outputs/1 -> [BSCP_outputs]
  BOUTP_outputs/1 -> [BOUTP_outputs]
  [CAN6_SysPowerMode] -> bus_creator/1  "CAN6_SysPowerMode"
  bus_creator/1 -> FD6_C200_0/1
  SysPowerMode/1(CAN6_SysPowerMode) -> [CAN6_SysPowerMode]
  bus_selector/1 -> SysPowerMode/1(SysPowerMode)  "<VOUTP_SysPowerMode_enum>"
  [BOUTP_outputs] -> bus_selector/1
